simulink model "gm_untitled"  (R2016b)
settings: Solver=FixedStepAuto  StartTime=0.0  StopTime=10.0  FixedStep=0.2  RelTol=1e-3
settings Model: ExtModeAutoUpdateStatusClock=off  Creator=hasee  LastModifiedBy=hasee
settings DataIOCC: LimitDataPoints=on  SaveOutput=off  SaveTime=off
settings OptimizationCC: BlockReduction=off  ConditionallyExecuteInputs=off  DefaultParameterBehavior=Inlined  ExpressionDepthLimit=2147483647  InitFltsAndDblsToZero=on  LifeSpan=inf
settings DebuggingCC: AlgebraicLoopMsg=error  SaveWithParameterizedLinksMsg=none  UnderspecifiedInitializationDetection=Classic  MergeDetectMultiDrivingBlocksExec=none  SignalResolutionControl=TryResolveAllWithWarning  InheritedTsInSrcMsg=none  MultiTaskDSMMsg=warning  MultiTaskCondExecSysMsg=none  SingleTaskRateTransMsg=error  FcnCallInpInsideContextMsg=warning  AllowSymbolicDim=off  StateNameClashWarn=warning  StrictBusMsg=ErrorOnBusTreatedAsVector  SFUnexpectedBacktrackingDiag=warning  SFNoUnconditionalDefaultTransitionDiag=warning  SFExecutionAtInitializationDiag=none
settings HardwareCC: ProdBitPerPointer=32  ProdBitPerSizeT=32  ProdBitPerPtrDiffT=32  ProdLargestAtomicFloat=None  ProdIntDivRoundTo=Undefined  ProdEndianess=Unspecified  ProdWordSize=32  ProdHWDeviceType=ASIC/FPGA->ASIC/FPGA  TargetHWDeviceType=32-bit Generic  ProdEqTarget=off
settings GRTTargetCC: TargetFcnLib=ansi_tfl_tmw.mat  TargetLangStandard=C89/C90 (ANSI)  GeneratePreprocessorConditionals=Disable all  CombineOutputUpdateFcns=off  GRTInterface=on
settings ConfigComp: CovScope=ReferencedModels  CovMetricSettings=dw  CovHtmlReporting=on  CovSaveCumulativeToWorkspaceVar=on  CovSaveSingleToWorkspaceVar=on  CovExternalEMLEnable=off  CovSFcnEnable=off

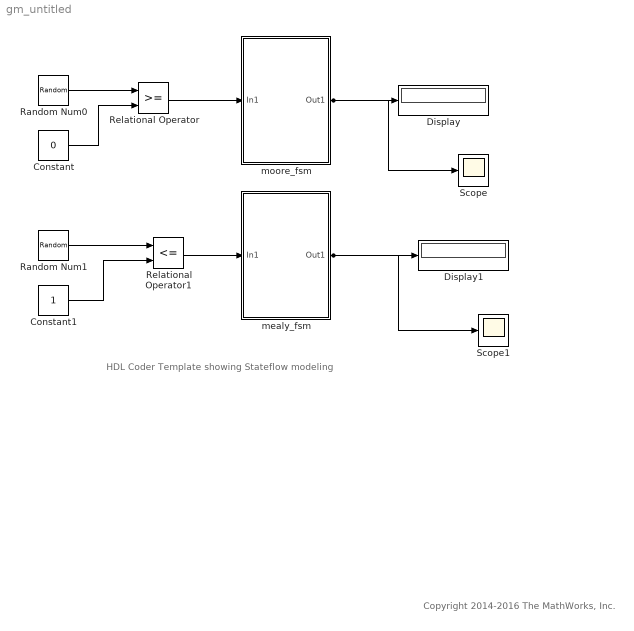
== system gm_untitled ==
  note: Copyright 2014-2016 The MathWorks, Inc.
  note: HDL Coder Template showing Stateflow modeling
  Constant : Constant  Value=0
  Constant1 : Constant
  Display : Display
  Display1 : Display
  Random Num0 : RandomNumber  SampleTime=0
  Random Num1 : RandomNumber  SampleTime=0
  Relational Operator : RelationalOperator  OutDataTypeStr=boolean  RndMeth=Nearest
  Relational Operator1 : RelationalOperator  Operator=<=  OutDataTypeStr=boolean  RndMeth=Nearest
  Scope : Scope
  Scope1 : Scope
  mealy_fsm : Subsystem
  moore_fsm : Subsystem
  wires:
  Relational Operator1/1 -> mealy_fsm/1(In1)
  Constant1/1 -> Relational Operator1/2
  Random Num1/1 -> Relational Operator1/1
  mealy_fsm/1(Out1) -> Scope1/1, Display1/1
  moore_fsm/1(Out1) -> Scope/1, Display/1
  Relational Operator/1 -> moore_fsm/1(In1)
  Constant/1 -> Relational Operator/2
  Random Num0/1 -> Relational Operator/1

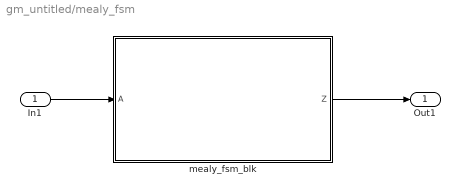
== system gm_untitled/mealy_fsm ==
  In1 : Inport
  mealy_fsm_blk : MATLAB Function  TreatAsAtomicUnit=on
  Out1 : Outport
  wires:
  mealy_fsm_blk/1(Z) -> Out1/1
  In1/1 -> mealy_fsm_blk/1(A)

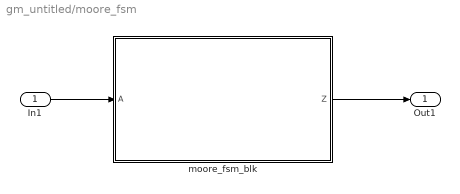
== system gm_untitled/moore_fsm ==
  In1 : Inport
  moore_fsm_blk : MATLAB Function  TreatAsAtomicUnit=on
  Out1 : Outport
  wires:
  In1/1 -> moore_fsm_blk/1(A)
  moore_fsm_blk/1(Z) -> Out1/1

== matlab function gm_untitled/mealy_fsm/mealy_fsm_blk ==
  settings: fimath=|
      | fimath(...
      | 'RoundMode', 'nearest',...
      | 'OverflowMode', 'saturate',...
      | 'ProductMode', 'FullPrecision', 'ProductWordLength', 128,...
      | 'SumMode', 'FullPrecision', 'SumWordLength', 128,...
      | 'CastBeforeSum', true)
  data: A input boolean; Z output boolean size=1
function Z = mealy_fsm(A)
% Mealy State Machine

% y = f(x,u) : 
% all actions are condition actions and 
% outputs are function of state and input 

persistent mealy_state_reg;
if isempty(mealy_state_reg)
    mealy_state_reg = fi(0, 0, 2, 0, hdlfimath);   
end

S1 = 0;
S2 = 1;
S3 = 2;
S4 = 3;

% switch to new state based on the value state register
switch (mealy_state_reg) 
    
    case S1,
        
        % value of output 'Z' depends both on state and inputs
        if (A)
            Z = true;
            mealy_state_reg(1) = S1;
        else
            Z = false;            
            mealy_state_reg(1) = S2;
        end
        
    case S2,
        
        if (A)
            Z = false;
            mealy_state_reg(1) = S1;
        else
            Z = true;
            mealy_state_reg(1) = S2;
        end
        
    case S3,
        
        if (A)
            Z = false;            
            mealy_state_reg(1) = S2;
        else
            Z = true;            
            mealy_state_reg(1) = S3;
        end
        
    case S4,
        
        if (A)
            Z = true;
            mealy_state_reg(1) = S1;
        else
            Z = false;            
            mealy_state_reg(1) = S3;
        end        
        
    otherwise,
        
        Z = false;
end

== matlab function gm_untitled/moore_fsm/moore_fsm_blk ==
  settings: fimath=|
      | fimath(...
      | 'RoundMode', 'nearest',...
      | 'OverflowMode', 'saturate',...
      | 'ProductMode', 'FullPrecision', 'ProductWordLength', 128,...
      | 'SumMode', 'FullPrecision', 'SumWordLength', 128,...
      | 'CastBeforeSum', true)
  data: A input boolean; Z output boolean size=1
function Z = moore_fsm(A)
% Moore State Machine

% y = f(x) : 
% all actions are state actions and 
% outputs are pure functions of state only 

% using persistent keyword to model state registers in hardware
persistent moore_state_reg;
if isempty(moore_state_reg)
    moore_state_reg = fi(0, 0, 2, 0, hdlfimath);   
end

S1 = 0;
S2 = 1;
S3 = 2;
S4 = 3;

% switch to new state based on the value state register
switch (moore_state_reg)
    
    case S1,
        
        % value of output 'Z' depends both only on state and not on inputs
        Z = true;
        
        % decide next state value based on inputs
        if (~A)
            moore_state_reg(1) = S1;
        else
            moore_state_reg(1) = S2;
        end
        
    case S2,
        
        Z = false;
        
        if (~A)
            moore_state_reg(1) = S1;
        else
            moore_state_reg(1) = S2;
        end
        
    case S3,
        
        Z = false;
        
        if (~A)
            moore_state_reg(1) = S2;
        else
            moore_state_reg(1) = S3;
        end
        
    case S4,
        
        Z = true;
        if (~A)
            moore_state_reg(1) = S1;
        else
            moore_state_reg(1) = S3;
        end
    otherwise,
        Z = false;
end
